simulink library "mach_lib"  (Simulink 6.3)
undefined symbols (not defined in the file): accel_cmd, aero_surf_qbar_off, aero_surf_qbar_on, altitude_stop, angular_rate_stop, att_cmd_select, att_trim_IC, att_type, att_type_numbers, bb_ellipsoid, bb_params, chi_trim_IC, command_time, compute_all_rate_cols, compute_all_vel_cols, constants, cosA, da_trim_IC, de_trim_IC, DiscIntNeverNeededParam, dr_trim_IC, dtsim, E_rwy, E_trim_IC, Ed_cmd, Ed_trim_IC, energy_stop, eow_boundary, full_surf_llim, full_surf_ulim, gain_var_struct, gam_cmd_descent, gam_cmd_preflare, gamdot_cmd_descent, gamdot_cmd_flare, gamdot_cmd_preflare, gamma_trim_IC, h_trim_IC, hd_cmd, hd_trim_IC, ideal_vel_Kb, integrate_start_time_sim, integrate_state_sim, llim, MACH, MACH_att_fb, MACH_gain_mat, MACH_mass_IC, MACH_pos_IC, MACH_pqr_Bmat_IC, MACH_pqr_IC, MACH_pqr_u_IC, MACH_quat_IC, MACH_throttle_IC, MACH_U_nom_IC, MACH_vel_Bmat_IC, MACH_vel_cvdnom_IC, MACH_vel_IC, MACH_vel_uold_IC, max_chi_cmd ... (+67)
libraries: simulink x75, mach_lib x27, utility_lib x25, model_lib x7, models x6
(part 4 of 6)

== system mach_lib/claw_main/grab ExportedGlobal/grab cv variables/Subsystem ==
  In1 : Inport
  In2 : Inport  Port=2
  In3 : Inport  Port=3
  In4 : Inport  Port=4
  In5 : Inport  Port=5
  In6 : Inport  Port=6
  In7 : Inport  Port=7
  In8 : Inport  Port=8
  In9 : Inport  Port=9
  In10 : Inport  Port=10
  In11 : Inport  Port=11
  In12 : Inport  Port=12
  In13 : Inport  Port=13
  Out1 : Outport
  Out2 : Outport  Port=2
  Out3 : Outport  Port=3
  Out4 : Outport  Port=4
  Out5 : Outport  Port=5
  Out6 : Outport  Port=6
  Out7 : Outport  Port=7
  Out8 : Outport  Port=8
  Out9 : Outport  Port=9
  Out10 : Outport  Port=10
  Out11 : Outport  Port=11
  Out12 : Outport  Port=12
  Out13 : Outport  Port=13
  wires:
  In13/1 -> Out13/1
  In12/1 -> Out12/1
  In11/1 -> Out11/1
  In10/1 -> Out10/1
  In9/1 -> Out9/1
  In8/1 -> Out8/1
  In7/1 -> Out7/1
  In6/1 -> Out6/1
  In5/1 -> Out5/1
  In4/1 -> Out4/1
  In3/1 -> Out3/1
  In2/1 -> Out2/1
  In1/1 -> Out1/1

== system mach_lib/claw_main/grab ExportedGlobal/grab cvcmd variables/Subsystem ==
  In1 : Inport
  In2 : Inport  Port=2
  In3 : Inport  Port=3
  In4 : Inport  Port=4
  In5 : Inport  Port=5
  In6 : Inport  Port=6
  In7 : Inport  Port=7
  In8 : Inport  Port=8
  In9 : Inport  Port=9
  In10 : Inport  Port=10
  In11 : Inport  Port=11
  In12 : Inport  Port=12
  In13 : Inport  Port=13
  Out1 : Outport
  Out2 : Outport  Port=2
  Out3 : Outport  Port=3
  Out4 : Outport  Port=4
  Out5 : Outport  Port=5
  Out6 : Outport  Port=6
  Out7 : Outport  Port=7
  Out8 : Outport  Port=8
  Out9 : Outport  Port=9
  Out10 : Outport  Port=10
  Out11 : Outport  Port=11
  Out12 : Outport  Port=12
  Out13 : Outport  Port=13
  wires:
  In13/1 -> Out13/1
  In12/1 -> Out12/1
  In11/1 -> Out11/1
  In10/1 -> Out10/1
  In9/1 -> Out9/1
  In8/1 -> Out8/1
  In7/1 -> Out7/1
  In6/1 -> Out6/1
  In5/1 -> Out5/1
  In4/1 -> Out4/1
  In3/1 -> Out3/1
  In2/1 -> Out2/1
  In1/1 -> Out1/1

== system mach_lib/claw_main/grab ExportedGlobal/grab cvdex variables/Subsystem ==
  In1 : Inport
  In2 : Inport  Port=2
  In3 : Inport  Port=3
  In4 : Inport  Port=4
  In5 : Inport  Port=5
  In6 : Inport  Port=6
  In7 : Inport  Port=7
  In8 : Inport  Port=8
  In9 : Inport  Port=9
  In10 : Inport  Port=10
  In11 : Inport  Port=11
  In12 : Inport  Port=12
  In13 : Inport  Port=13
  Out1 : Outport
  Out2 : Outport  Port=2
  Out3 : Outport  Port=3
  Out4 : Outport  Port=4
  Out5 : Outport  Port=5
  Out6 : Outport  Port=6
  Out7 : Outport  Port=7
  Out8 : Outport  Port=8
  Out9 : Outport  Port=9
  Out10 : Outport  Port=10
  Out11 : Outport  Port=11
  Out12 : Outport  Port=12
  Out13 : Outport  Port=13
  wires:
  In13/1 -> Out13/1
  In12/1 -> Out12/1
  In11/1 -> Out11/1
  In10/1 -> Out10/1
  In9/1 -> Out9/1
  In8/1 -> Out8/1
  In7/1 -> Out7/1
  In6/1 -> Out6/1
  In5/1 -> Out5/1
  In4/1 -> Out4/1
  In3/1 -> Out3/1
  In2/1 -> Out2/1
  In1/1 -> Out1/1

== system mach_lib/claw_main/grab ExportedGlobal/grab integrator variables/Subsystem ==
  In1 : Inport
  In2 : Inport  Port=2
  In3 : Inport  Port=3
  In4 : Inport  Port=4
  In5 : Inport  Port=5
  In6 : Inport  Port=6
  In7 : Inport  Port=7
  In8 : Inport  Port=8
  In9 : Inport  Port=9
  In10 : Inport  Port=10
  In11 : Inport  Port=11
  In12 : Inport  Port=12
  In13 : Inport  Port=13
  Out1 : Outport
  Out2 : Outport  Port=2
  Out3 : Outport  Port=3
  Out4 : Outport  Port=4
  Out5 : Outport  Port=5
  Out6 : Outport  Port=6
  Out7 : Outport  Port=7
  Out8 : Outport  Port=8
  Out9 : Outport  Port=9
  Out10 : Outport  Port=10
  Out11 : Outport  Port=11
  Out12 : Outport  Port=12
  Out13 : Outport  Port=13
  wires:
  In13/1 -> Out13/1
  In12/1 -> Out12/1
  In11/1 -> Out11/1
  In10/1 -> Out10/1
  In9/1 -> Out9/1
  In8/1 -> Out8/1
  In7/1 -> Out7/1
  In6/1 -> Out6/1
  In5/1 -> Out5/1
  In4/1 -> Out4/1
  In3/1 -> Out3/1
  In2/1 -> Out2/1
  In1/1 -> Out1/1

== system mach_lib/claw_main/grab ExportedGlobal/grab w_est variables/Subsystem ==
  In1 : Inport
  In2 : Inport  Port=2
  In3 : Inport  Port=3
  Out1 : Outport
  Out2 : Outport  Port=2
  Out3 : Outport  Port=3
  wires:
  In3/1 -> Out3/1
  In2/1 -> Out2/1
  In1/1 -> Out1/1

== system mach_lib/claw_main/input processing/mode dependent stick processing/att rate cmd ==
  note: In attitude, velocity, position mode, while enabled,
      | replace cam command with integrated rate command.
      |
      | In attitude mode, while enabled,
      | replace the other att commands with integrated rate commands.
      |
      | integrators are set to current values upon transition into this condition.
      | Reset of cam cmd can be disabled by setting
      | reset_camcmd_on_entry to false.
      |
      | In addition to specified conditions, reset also occurs, if applicable
      | when att_type changes
  mode : Inport
  command_in : Inport  Port=2
  signal_bus : Inport  Port=3
  Bus Selector3 : BusSelector  OutputSignals=mode_sw.att_rate_cmd_sw,mode_sw.cam_rate_cmd_sw,y_meas.dircos
  Compare To Constant1 : simulink/Logic and Bit Operations/Compare To Constant  relop===  const=modes.att  LogicOutDataTypeMode=boolean  ZeroCross=off
  Compare To Constant2 : simulink/Logic and Bit Operations/Compare To Constant  relop=>=  const=modes.att  LogicOutDataTypeMode=boolean  ZeroCross=off
  Gain1 : Gain  Gain=[ 1 1 reset_camcmd_on_entry ]
  Logical Operator1 : Logic  Operator=OR  AllPortsSameDT=off
  Logical Operator2 : Logic  AllPortsSameDT=off
  Logical Operator4 : Logic  AllPortsSameDT=off
  Multiport Switch1 : MultiPortSwitch  Inputs=2  zeroidx=on
  Mux : Mux  Inputs=3
  Product1 : Product  RndMeth=Zero
  also reset att on att_type change : Subsystem
  att cmd integration : DiscreteIntegrator  ExternalReset=either  InitialConditionSource=external  SampleTime=-1  ICPrevOutput=DiscIntNeverNeededParam  ICPrevScaledInput=DiscIntNeverNeededParam
  att/att rate cmd : Selector  Elements=1:3  InputPortWidth=4
  dc2att : utility_lib/dc2att
  set att cmd : Assignment  Elements=1:3  OutputInitialize=Initialize using input (U1)
  command_out : Outport
  wires:
  Bus Selector3/3 -> dc2att/1  "<dircos>"
  Bus Selector3/2 -> Logical Operator1/2  "<cam_rate_cmd_sw>"
  Bus Selector3/1 -> Logical Operator1/1, Logical Operator4/2  "<att_rate_cmd_sw>"
  signal_bus/1 -> Bus Selector3/1
  dc2att/1 -> att cmd integration/3
  set att cmd/1 -> command_out/1
  Multiport Switch1/1 -> set att cmd/2
  Mux/1 -> Multiport Switch1/1, also reset att on att_type change/1(reset_in), Product1/2
  Compare To Constant2/1 -> Logical Operator2/2
  Logical Operator2/1 -> Mux/3
  Logical Operator1/1 -> Logical Operator2/1
  Logical Operator4/1 -> Mux/2, Mux/1
  att/att rate cmd/1 -> Multiport Switch1/2, Product1/1
  Compare To Constant1/1 -> Logical Operator4/1
  command_in/1 -> att/att rate cmd/1, set att cmd/1
  mode/1 -> Compare To Constant2/1, Compare To Constant1/1
  also reset att on att_type change/1(reset_out) -> Gain1/1
  att cmd integration/1 -> Multiport Switch1/3
  Gain1/1 -> att cmd integration/2
  Product1/1 -> att cmd integration/1

== system mach_lib/claw_main/input processing/mode dependent stick processing/att_type cmd ==
  mode : Inport
  command_in : Inport  Port=2
  signal_bus : Inport  Port=3
  Bus Selector3 : BusSelector  OutputSignals=mode_sw.att_type
  Compare To Constant1 : simulink/Logic and Bit Operations/Compare To Constant  relop===  const=modes.att  LogicOutDataTypeMode=boolean  ZeroCross=off
  Constant4 : Constant  Value=use_auto_att_type
  From Workspace1 : FromWorkspace  VariableName=rpy_cmd_fw  SampleTime=MACH.dt  OutputAfterFinalValue=Holding final value
  From Workspace2 : FromWorkspace  VariableName=mab_cmd_fw  SampleTime=MACH.dt  OutputAfterFinalValue=Holding final value
  From Workspace4 : FromWorkspace  VariableName=tiltcam_cmd_fw  SampleTime=MACH.dt  OutputAfterFinalValue=Holding final value
  Logical Operator4 : Logic  AllPortsSameDT=off
  Multiport Switch1 : MultiPortSwitch  Inputs=2  zeroidx=on
  Multiport Switch2 : MultiPortSwitch  Inputs=length(att_type_numbers)
  att cmd : Selector  Elements=1:3  InputPortWidth=4
  bam_cmd : Selector  Elements=[3 2 1]  InputPortWidth=3
  set att cmd : Assignment  Elements=1:3  OutputInitialize=Initialize using input (U1)
  ypr_cmd : Selector  Elements=[3 2 1]  InputPortWidth=3
  command_out : Outport
  wires:
  ypr_cmd/1 -> Multiport Switch2/4
  Multiport Switch2/1 -> Multiport Switch1/3
  bam_cmd/1 -> Multiport Switch2/6
  From Workspace1/1 -> ypr_cmd/1, Multiport Switch2/3
  From Workspace2/1 -> bam_cmd/1, Multiport Switch2/5
  From Workspace4/1 -> Multiport Switch2/2
  Bus Selector3/1 -> Multiport Switch2/1  "<att_type>"
  Constant4/1 -> Logical Operator4/2
  mode/1 -> Compare To Constant1/1
  command_in/1 -> set att cmd/1, att cmd/1
  Compare To Constant1/1 -> Logical Operator4/1
  att cmd/1 -> Multiport Switch1/2
  Logical Operator4/1 -> Multiport Switch1/1
  Multiport Switch1/1 -> set att cmd/2
  set att cmd/1 -> command_out/1
  signal_bus/1 -> Bus Selector3/1

== system mach_lib/claw_main/input processing/mode dependent stick processing/feed forward ==
  table_bus : Inport
  signal_bus : Inport  Port=2
  Bus Creator : BusCreator
  Bus Selector : BusSelector  OutputSignals=eow_idx,eow_large,X_idx
  Constant : Constant  Value=use_eow_as_iv
  Constant1 : Constant  Value=zeros(MACH.pqr_num_cv,1)
  From Workspace1 : FromWorkspace  VariableName=vel_ff_fw  SampleTime=MACH.dt  OutputAfterFinalValue=Holding final value
  From Workspace4 : FromWorkspace  VariableName=pos_ff_fw  SampleTime=MACH.dt  OutputAfterFinalValue=Holding final value
  Switch{,1..3} (4 alike) : Switch  Threshold=0.5
  get att_ff : Subsystem
  lookup using  energy over weight : Subsystem
  "lookup using X  " : Subsystem
  feed_forward : Outport
  wires:
  signal_bus/1 -> get att_ff/1(signal_bus)
  Bus Selector/3 -> "lookup using X  "/1(X_idx)  "<X_idx>"
  Bus Selector/2 -> Switch3/2, Switch2/2  "<eow_large>"
  Bus Selector/1 -> lookup using  energy over weight/1(eow_idx)  "<eow_idx>"
  table_bus/1 -> Bus Selector/1
  "lookup using X  "/1(pos_ff) -> Switch2/3
  "lookup using X  "/2(vel_ff) -> Switch3/3
  lookup using  energy over weight/2(vel_ff) -> Switch3/1
  Switch3/1 -> Switch1/1
  lookup using  energy over weight/1(pos_ff) -> Switch2/1
  Switch2/1 -> Switch/1
  Constant/1 -> Switch/2, Switch1/2
  From Workspace1/1 -> Switch1/3
  From Workspace4/1 -> Switch/3
  Bus Creator/1 -> feed_forward/1
  Constant1/1 -> Bus Creator/4  "pqr_ff"
  get att_ff/1(att_ff) -> Bus Creator/3  "att_ff"
  Switch1/1 -> Bus Creator/2  "vel_ff"
  Switch/1 -> Bus Creator/1  "pos_ff"

== system mach_lib/claw_main/input processing/mode dependent stick processing/llh cmd ==
  mode : Inport
  command_in : Inport  Port=2
  signal_bus : Inport  Port=3
  Assignment : Assignment  Elements=[1 2 4]  OutputInitialize=Initialize using input (U1)
  Bus Selector : BusSelector  OutputSignals=mode_sw.llh_input_sw,y_meas.vehicle_origin
  Compare To Constant1 : simulink/Logic and Bit Operations/Compare To Constant  relop===  const=modes.pos  LogicOutDataTypeMode=boolean  ZeroCross=off
  LLh2NEh : utility_lib/LLh2NEh
  Logical Operator4 : Logic  AllPortsSameDT=off
  Multiport Switch2 : MultiPortSwitch  Inputs=2  zeroidx=on  SaturateOnIntegerOverflow=on
  Selector1 : Selector  Elements=[1 2 4]  InputPortWidth=4
  command_out : Outport
  wires:
  mode/1 -> Compare To Constant1/1
  Logical Operator4/1 -> Multiport Switch2/1
  Bus Selector/1 -> Logical Operator4/2  "<llh_input_sw>"
  Compare To Constant1/1 -> Logical Operator4/1
  signal_bus/1 -> Bus Selector/1
  Multiport Switch2/1 -> command_out/1
  Assignment/1 -> Multiport Switch2/3
  LLh2NEh/1 -> Assignment/2
  Selector1/1 -> LLh2NEh/1
  command_in/1 -> Selector1/1, Assignment/1, Multiport Switch2/2
  Bus Selector/2 -> LLh2NEh/2  "<vehicle_origin>"

== system mach_lib/claw_main/input processing/mode dependent stick processing/rampin vel_cmd ==
  mode : Inport
  command_in : Inport  Port=2
  NEh_dot : Inport  Port=3
  Compare To Constant : simulink/Logic and Bit Operations/Compare To Constant  relop=<=  const=modes.att  LogicOutDataTypeMode=boolean  ZeroCross=off
  Compare To Constant1 : simulink/Logic and Bit Operations/Compare To Constant  relop===  const=modes.vel  LogicOutDataTypeMode=boolean  ZeroCross=off
  Constant : Constant  Value=MACH.dt/max(vel_cmd_ramp_time,MACH.dt)
  Constant1 : Constant
  Constant2 : Constant  Value=0
  Logical Operator : Logic  AllPortsSameDT=off
  MinMax : MinMax  Function=max  Inputs=2
  Product : Product  RndMeth=Zero
  Product1 : Product  RndMeth=Zero
  Sum : Sum  Inputs=-+|
  Sum2 : Sum  Inputs=|++
  Sum3 : Sum  Inputs=|+-
  Switch : Switch  Threshold=0.5
  Switch1 : Switch  Threshold=0.5
  Unit Delay : UnitDelay  Orientation=left  SampleTime=-1
  Unit Delay1 : UnitDelay  SampleTime=-1
  Unit Delay2 : UnitDelay  Orientation=left  SampleTime=-1
  set vel cmd : Assignment  Elements=[1 2 4]  OutputInitialize=Initialize using input (U1)
  vel cmd : Selector  Elements=[1 2 4]  InputPortWidth=4
  command_out : Outport
  wires:
  Constant2/1 -> MinMax/1
  MinMax/1 -> Unit Delay2/1, Product/2
  Constant/1 -> Sum3/2
  Sum3/1 -> MinMax/2
  Product/1 -> Sum2/2
  Switch1/1 -> Sum3/1
  Constant1/1 -> Switch1/1
  Product1/1 -> Switch1/3
  Sum2/1 -> set vel cmd/2
  command_in/1 -> vel cmd/1, set vel cmd/1
  vel cmd/1 -> Sum/1, Sum2/1
  set vel cmd/1 -> command_out/1
  Sum/1 -> Switch/1
  NEh_dot/1 -> Sum/2
  Switch/1 -> Product/1, Unit Delay/1
  Unit Delay/1 -> Switch/3
  mode/1 -> Compare To Constant1/1, Unit Delay1/1
  Unit Delay1/1 -> Compare To Constant/1
  Compare To Constant/1 -> Logical Operator/1
  Compare To Constant1/1 -> Product1/1, Logical Operator/2
  Logical Operator/1 -> Switch1/2, Switch/2
  Unit Delay2/1 -> Product1/2

== system mach_lib/claw_main/input processing/mode dependent stick processing/set command selection switches ==
  accel_cmd_sw : Inport
  CLAW_mode : Inport  Port=2
  Bus Creator : BusCreator
  Constant : Constant  Value=MACH.select_cmd_array
  Demux : Demux  Outputs=[4 5 4 4]
  Reshape : simulink/Math Operations/Reshape  OutputDimensionality=1-D array  OutputDimensions=[1,1]
  Selector : Selector  InputType=Matrix  IndexMode=Zero-based  Elements=[1 3]  Rows=-1  ColumnSrc=External  InputPortWidth=3
  modify for accel cmd submode : Subsystem
  select_cmd : Outport
  wires:
  accel_cmd_sw/1 -> modify for accel cmd submode/2(accel_cmd_sw)
  Bus Creator/1 -> modify for accel cmd submode/1(select_cmd_in)
  modify for accel cmd submode/1(select_cmd) -> select_cmd/1
  Reshape/1 -> Demux/1
  Demux/4 -> Bus Creator/4  "pos"
  Demux/3 -> Bus Creator/3  "vel"
  Demux/2 -> Bus Creator/2  "att"
  Demux/1 -> Bus Creator/1  "rate"
  Selector/1 -> Reshape/1
  CLAW_mode/1 -> Selector/2
  Constant/1 -> Selector/1

== system mach_lib/claw_main/input processing/mode dependent stick processing/table iv computation ==
  x_est : Inport
  Bus Creator : BusCreator  Inputs=5
  Compare To Constant : simulink/Logic and Bit Operations/Compare To Constant  relop=>=  const=eow_boundary  LogicOutDataTypeMode=boolean  ZeroCross=off
  Constant : Constant  Value=2*constants.g
  Constant1 : Constant  Value=sinA
  Constant2 : Constant  Value=cosA
  Constant3 : Constant  Value=N_rwy
  Constant4 : Constant  Value=E_rwy
  Dot Product : simulink/Math Operations/Dot Product  InputSameDT=on  OutDataType=sfix(16)  OutScaling=2^-10  DoSatur=off
  PreLookup Index Search : simulink/Lookup Tables/PreLookup Index Search  bpData=tbl_eow  searchMode=Binary Search  cacheBpFlag=off  outputFlag=off  IndexDataType=uint32  extrapMode=Linear Extrapolation  rangeErrorMode=None
  PreLookup Index Search1 : simulink/Lookup Tables/PreLookup Index Search  bpData=tbl_X  searchMode=Binary Search  cacheBpFlag=off  outputFlag=off  IndexDataType=uint32  extrapMode=Clip to Range  rangeErrorMode=None
  Product1 : Product  RndMeth=Zero
  Product2 : Product  Inputs=*/  RndMeth=Zero
  Product3 : Product  RndMeth=Zero
  Sum1 : Sum  Inputs=|++
  Sum2 : Sum  Inputs=-+|
  Sum3 : Sum  Inputs=+|+
  Sum4 : Sum  Inputs=|+-
  get E : Selector  Elements=8  InputPortWidth=13
  get N : Selector  Elements=7  InputPortWidth=13
  get h : Selector  Elements=9  InputPortWidth=13
  get uvw : Selector  Elements=4:6  InputPortWidth=13
  table_bus : Outport
  wires:
  Compare To Constant/1 -> Bus Creator/1  "eow_large"
  PreLookup Index Search1/1 -> Bus Creator/5  "X_idx"
  Bus Creator/1 -> table_bus/1
  Sum3/1 -> Bus Creator/4, PreLookup Index Search1/1  "X"
  Sum4/1 -> Product1/2
  Constant4/1 -> Sum4/2
  Constant3/1 -> Sum2/1
  Constant1/1 -> Product1/1
  Product1/1 -> Sum3/2
  get E/1 -> Sum4/1
  Constant2/1 -> Product3/2
  Product3/1 -> Sum3/1
  Sum2/1 -> Product3/1
  get N/1 -> Sum2/2
  PreLookup Index Search/1 -> Bus Creator/3  "eow_idx"
  Sum1/1 -> Bus Creator/2, Compare To Constant/1, PreLookup Index Search/1  "eow"
  x_est/1 -> get E/1, get N/1, get uvw/1, get h/1
  Product2/1 -> Sum1/2
  Dot Product/1 -> Product2/1
  Constant/1 -> Product2/2
  get h/1 -> Sum1/1
  get uvw/1 -> Dot Product/2, Dot Product/1

== system mach_lib/claw_main/input processing/mode dependent stick processing/use table lookup pos cmds ==
  mode : Inport
  command_in : Inport  Port=2
  table_bus : Inport  Port=3
  Assertion : Assertion  Enabled=off  AssertionFailFcn=assertioncb  StopWhenAssertionFail=off
  Bus Selector : BusSelector  OutputSignals=eow_idx,eow_large,X_idx,X
  Compare To Constant1 : simulink/Logic and Bit Operations/Compare To Constant  relop===  const=modes.pos  LogicOutDataTypeMode=boolean  ZeroCross=off
  Constant4 : Constant  Value=use_eow_as_iv
  Logical Operator : Logic  AllPortsSameDT=off
  Relational Operator : RelationalOperator  LogicOutDataTypeMode=Boolean
  Switch1 : Switch  Threshold=0.5
  Switch2 : Switch  Threshold=0.5
  Unit Delay : UnitDelay  SampleTime=-1
  pos cmd : Selector  Elements=[1 2 4]  InputPortWidth=4
  set pos cmd : Assignment  Elements=[1 2 4]  OutputInitialize=Initialize using input (U1)
  use E/W to get pos cmds : Subsystem
  use X to get pos cmds : Subsystem
  command_out : Outport
  wires:
  Relational Operator/1 -> Assertion/1
  Unit Delay/1 -> Relational Operator/1
  Bus Selector/4 -> use X to get pos cmds/2(X)  "<X>"
  Bus Selector/3 -> use X to get pos cmds/1(X_idx)  "<X_idx>"
  Bus Selector/1 -> use E/W to get pos cmds/1(eow_idx)  "<eow_idx>"
  table_bus/1 -> Bus Selector/1
  Bus Selector/2 -> Switch1/2  "<eow_large>"
  Switch1/1 -> Switch2/1
  use X to get pos cmds/1(pos_cmd_X) -> Switch1/3
  use E/W to get pos cmds/1(pos_cmd_eow) -> Switch1/1
  Switch2/1 -> set pos cmd/2
  command_in/1 -> pos cmd/1, set pos cmd/1
  pos cmd/1 -> Switch2/3
  set pos cmd/1 -> command_out/1
  mode/1 -> Compare To Constant1/1
  Constant4/1 -> Logical Operator/1
  Compare To Constant1/1 -> Logical Operator/2
  Logical Operator/1 -> Relational Operator/2, Unit Delay/1, Switch2/2

== system mach_lib/claw_main/input processing/modify limits and apply to direct commands/apply surface locking ==
  u_meas : Inport
  full_surf_in : Inport  Port=2
  Bus Assignment : BusAssignment  AssignedSignals=full_surf_ulim,full_surf_llim
  Bus Selector : BusSelector  OutputSignals=full_surf_ulim,full_surf_cmd,full_surf_lock,full_surf_llim
  Multiport Switch : MultiPortSwitch  Inputs=3  zeroidx=on
  Multiport Switch1 : MultiPortSwitch  Inputs=3  zeroidx=on
  full_surf : Outport
  wires:
  Bus Selector/4 -> Multiport Switch1/2  "<full_surf_llim>"
  Bus Selector/2 -> Multiport Switch1/3, Multiport Switch/3  "<full_surf_cmd>"
  Bus Selector/1 -> Multiport Switch/2  "<full_surf_ulim>"
  Bus Selector/3 -> Multiport Switch/1, Multiport Switch1/1  "<full_surf_lock>"
  Bus Assignment/1 -> full_surf/1
  u_meas/1 -> Multiport Switch/4, Multiport Switch1/4
  Multiport Switch1/1 -> Bus Assignment/3
  Multiport Switch/1 -> Bus Assignment/2
  full_surf_in/1 -> Bus Assignment/1, Bus Selector/1

== system mach_lib/claw_main/input processing/modify limits and apply to direct commands/throt out of fuel limits ==
  full_surf_in : Inport
  Bus Assignment : BusAssignment  AssignedSignals=full_surf_ulim,full_surf_llim
  Bus Selector3 : BusSelector  OutputSignals=full_surf_ulim,full_surf_llim
  throt out of fuel limits : model_lib/throt out of fuel limits
  full_surf : Outport
  wires:
  throt out of fuel limits/2 -> Bus Assignment/3
  throt out of fuel limits/1 -> Bus Assignment/2
  Bus Assignment/1 -> full_surf/1
  full_surf_in/1 -> Bus Assignment/1, Bus Selector3/1
  Bus Selector3/2 -> throt out of fuel limits/2  "<full_surf_llim>"
  Bus Selector3/1 -> throt out of fuel limits/1  "<full_surf_ulim>"

== system mach_lib/claw_main/input processing/select att_type/add tiebreaker for current att_type ==
  att_type_selected : Inport
  priority_in : Inport  Port=2
  Assignment1 : Assignment  IndexMode=Zero-based  ElementSrc=External  OutputInitialize=Initialize using input (U1)  OutputDimensions=length(att_type_numbers)+1
  Constant1 : Constant  Value=0.5
  Selector : Selector  IndexMode=Zero-based  ElementSrc=External  Elements=[1 3]  InputPortWidth=length(att_type_numbers)+1
  Sum1 : Sum  Inputs=|++
  Unit Delay : UnitDelay  SampleTime=-1
  priority_out : Outport
  wires:
  Assignment1/1 -> priority_out/1
  Unit Delay/1 -> Assignment1/3, Selector/2
  Sum1/1 -> Assignment1/2
  Constant1/1 -> Sum1/2
  Selector/1 -> Sum1/1
  priority_in/1 -> Assignment1/1, Selector/1
  att_type_selected/1 -> Unit Delay/1

== system mach_lib/claw_main/input processing/select att_type/compute precond vars ==
  signal_bus : Inport
  scoped_bus : Inport  Port=2
  -sin_b : Selector  InputPortWidth=9
  -sin_theta : Selector  Elements=7  InputPortWidth=9
  Bus Creator : BusCreator  Inputs=6
  Bus Selector2 : BusSelector  OutputSignals=aero_env_est.qbar,aero_env_est.vel,aero_env_est.beta,y_meas.dircos
  Bus Selector4 : BusSelector  OutputSignals=dc_L2W
  Saturation : Saturate  UpperLimit=1  LowerLimit=-1
  Saturation1 : Saturate  UpperLimit=1  LowerLimit=-1
  Trigonometric Function : Trigonometry  Operator=cos
  abs_cos_b : Fcn  Expr=sqrt(1-u(1)^2)
  abs_cos_beta : Abs
  abs_cos_gamma_rw : Abs
  abs_cos_theta : Fcn  Expr=sqrt(1-u(1)^2)
  abs_vel_rw : Abs
  cos_gamma_rw : Selector  Elements=9  InputPortWidth=9
  precond_vars : Outport
  wires:
  scoped_bus/1 -> Bus Selector4/1
  Bus Creator/1 -> precond_vars/1
  signal_bus/1 -> Bus Selector2/1
  Saturation1/1 -> abs_cos_b/1
  Saturation/1 -> abs_cos_theta/1
  abs_cos_gamma_rw/1 -> Bus Creator/6  "abs_cos_gamma_rw"
  abs_cos_b/1 -> Bus Creator/5  "abs_cos_b"
  abs_cos_theta/1 -> Bus Creator/4  "abs_cos_theta"
  abs_cos_beta/1 -> Bus Creator/3  "abs_cos_beta"
  abs_vel_rw/1 -> Bus Creator/2  "abs_vel_rw"
  cos_gamma_rw/1 -> abs_cos_gamma_rw/1
  -sin_theta/1 -> Saturation/1
  -sin_b/1 -> Saturation1/1
  Trigonometric Function/1 -> abs_cos_beta/1
  Bus Selector2/4 -> -sin_b/1, -sin_theta/1  "<dircos>"
  Bus Selector2/3 -> Trigonometric Function/1  "<beta>"
  Bus Selector2/2 -> abs_vel_rw/1  "<vel>"
  Bus Selector2/1 -> Bus Creator/1  "<qbar>"
  Bus Selector4/1 -> cos_gamma_rw/1  "<dc_L2W>"

== system mach_lib/claw_main/input processing/select att_type/evaluate preconditions ==
  precond_vars : Inport
  Bus Selector5 : BusSelector  OutputSignals=abs_cos_b,abs_cos_theta,abs_vel_rw,abs_cos_beta,abs_cos_gamma_rw,qbar
  Compare To Constant : simulink/Logic and Bit Operations/Compare To Constant  relop=>=  const=1  LogicOutDataTypeMode=boolean  ZeroCross=off
  Compare To Constant1 : simulink/Logic and Bit Operations/Compare To Constant  relop=>=  const=cos(pi/3)  LogicOutDataTypeMode=boolean  ZeroCross=off
  Compare To Constant2 : simulink/Logic and Bit Operations/Compare To Constant  relop=>=  const=0.1  LogicOutDataTypeMode=boolean  ZeroCross=off
  Compare To Constant3 : simulink/Logic and Bit Operations/Compare To Constant  relop=>=  const=cos(pi/3)  LogicOutDataTypeMode=boolean  ZeroCross=off
  Compare To Constant4 : simulink/Logic and Bit Operations/Compare To Constant  relop=>=  const=cos(pi/3)  LogicOutDataTypeMode=boolean  ZeroCross=off
  Compare To Constant5 : simulink/Logic and Bit Operations/Compare To Constant  relop=>=  const=1  LogicOutDataTypeMode=boolean  ZeroCross=off
  Constant : Constant  Value=boolean(0)
  Logical Operator : Logic  Inputs=4  AllPortsSameDT=off  OutDataTypeMode=Boolean
  Mux : Mux  Inputs=6
  precond_satisfied : Outport
  wires:
  Mux/1 -> precond_satisfied/1
  precond_vars/1 -> Bus Selector5/1
  Bus Selector5/6 -> Compare To Constant5/1  "<qbar>"
  Compare To Constant5/1 -> Logical Operator/4
  Constant/1 -> Mux/1
  Logical Operator/1 -> Mux/6, Mux/5
  Bus Selector5/5 -> Compare To Constant2/1  "<abs_cos_gamma_rw>"
  Bus Selector5/4 -> Compare To Constant1/1  "<abs_cos_beta>"
  Bus Selector5/3 -> Compare To Constant/1  "<abs_vel_rw>"
  Bus Selector5/2 -> Compare To Constant3/1  "<abs_cos_theta>"
  Bus Selector5/1 -> Compare To Constant4/1  "<abs_cos_b>"
  Compare To Constant4/1 -> Mux/2
  Compare To Constant3/1 -> Mux/4, Mux/3
  Compare To Constant2/1 -> Logical Operator/3
  Compare To Constant1/1 -> Logical Operator/2
  Compare To Constant/1 -> Logical Operator/1

== system mach_lib/claw_main/input processing/select att_type/select best att_type ==
  vec : Inport
  Constant4 : Constant  Value=0:length(att_type_numbers)
  Constant5 : Constant  Value=length(att_type_numbers)
  MinMax3 : MinMax  Function=max  SaturateOnIntegerOverflow=on  InputSameDT=on
  MinMax4 : MinMax  SaturateOnIntegerOverflow=on  InputSameDT=on
  Sum2 : Sum  Inputs=+-|  SaturateOnIntegerOverflow=on
  argmax1 : Switch  Threshold=-eps  SaturateOnIntegerOverflow=on
  idx_max : Outport
  wires:
  MinMax4/1 -> idx_max/1
  MinMax3/1 -> Sum2/2
  argmax1/1 -> MinMax4/1
  Constant5/1 -> argmax1/3
  Constant4/1 -> argmax1/1
  Sum2/1 -> argmax1/2
  vec/1 -> Sum2/1, MinMax3/1

== system mach_lib/claw_main/input processing/set control parameters/accel submode setup ==
  signal_bus : Inport
  Bus Selector1 : BusSelector  OutputSignals=mode_sw.enable_homing_sw,mode_sw.accel_submode,mode_sw.CLAW_mode
  Constant1 : Constant  Value=3
  Constant2 : Constant  Value=0
  Merge1 : Merge  Inputs=3  InitialOutput=zeros(3,1)
  Merge2 : Merge  Inputs=3  InitialOutput=zeros(3,1)
  NED_dd/vchigam_dot : Subsystem  TreatAsAtomicUnit=on
  Switch : Switch  Threshold=0.5
  Switch Case : SwitchCase  CaseConditions={[1 2],3}
  Switch1 : Switch  Threshold=0.5  InputSameDT=on
  homing : Subsystem  TreatAsAtomicUnit=on
  normal vel desdyn : Subsystem  TreatAsAtomicUnit=on
  accel_cmd_sw : Outport
  accel_cmd : Outport  Port=2
  wires:
  signal_bus/1 -> homing/1(signal_bus), NED_dd/vchigam_dot/2(signal_bus), Bus Selector1/1
  Constant2/1 -> Switch1/3
  Bus Selector1/3 -> Switch1/2  "<CLAW_mode>"
  normal vel desdyn/1(accel_cmd_sw) -> Merge2/3
  homing/1(accel_cmd_sw) -> Merge2/2
  homing/2(accel_cmd) -> Merge1/2
  NED_dd/vchigam_dot/2(accel_cmd) -> Merge1/1
  normal vel desdyn/2(accel_cmd) -> Merge1/3
  NED_dd/vchigam_dot/1(accel_cmd_sw) -> Merge2/1
  Merge2/1 -> accel_cmd_sw/1
  Merge1/1 -> accel_cmd/1
  Switch Case/3 -> normal vel desdyn/Action
  Switch Case/2 -> homing/Action
  Switch Case/1 -> NED_dd/vchigam_dot/Action
  Switch1/1 -> NED_dd/vchigam_dot/1(case), Switch Case/1
  Switch/1 -> Switch1/1
  Bus Selector1/2 -> Switch/3  "<accel_submode>"
  Bus Selector1/1 -> Switch/2  "<enable_homing_sw>"
  Constant1/1 -> Switch/1

== system mach_lib/claw_main/input processing/set control parameters/modify MACH_att_Kf ==
  gain_bus_in : Inport
  signal_bus : Inport  Port=2
  Bus Assignment : BusAssignment  AssignedSignals=MACH_att_Kf
  Bus Selector : BusSelector  OutputSignals=mode_sw.att_type
  Bus Selector1 : BusSelector  OutputSignals=MACH_att_Kf
  Compare To Constant : simulink/Logic and Bit Operations/Compare To Constant  relop=>=  const=att_type.mba_bank  LogicOutDataTypeMode=boolean  ZeroCross=off
  Constant : Constant  Value=MACH_att_fb
  Logical Operator : Logic  AllPortsSameDT=off
  Logical Operator1 : Logic  Operator=OR  AllPortsSameDT=off  OutDataTypeMode=Boolean
  Logical Operator2 : Logic  Operator=NOT  AllPortsSameDT=off  OutDataTypeMode=Boolean
  Logical Operator3 : Logic  AllPortsSameDT=off  OutDataTypeMode=Boolean
  gain_bus : Outport
  wires:
  Bus Assignment/1 -> gain_bus/1
  Logical Operator/1 -> Bus Assignment/2
  Logical Operator1/1 -> Logical Operator/2
  Compare To Constant/1 -> Logical Operator3/2
  Logical Operator3/1 -> Logical Operator1/2
  Bus Selector/1 -> Compare To Constant/1  "<att_type>"
  signal_bus/1 -> Bus Selector/1
  gain_bus_in/1 -> Bus Selector1/1, Bus Assignment/1
  Logical Operator2/1 -> Logical Operator1/1
  Constant/1 -> Logical Operator3/1, Logical Operator2/1
  Bus Selector1/1 -> Logical Operator/1  "<MACH_att_Kf>"

== system mach_lib/claw_main/input processing/set control parameters/select gains ==
  note: Note: Current variable gain structure will use gain_set = 1
      | if it exists, when enable_bb is true, otherwise gain_set = 0
      | (which is the global or selected default)
  enable_bb : Inport
  gain_set_in : Inport  Port=2
  Constant2 : Constant  Value=MACH_gain_mat
  MinMax : MinMax  Inputs=2
  Product : Product  Inputs=*/  RndMeth=Zero
  Reshape : simulink/Math Operations/Reshape  OutputDimensionality=1-D array  OutputDimensions=[1,1]
  Switch : Switch
  Width1 : Width
  Width2 : Width
  mux to bus : Subsystem  mask{var_struct=gain_var_struct}
      mask prompts: var_struct "var struct"
      mask init:
      | if(~isstruct(var_struct) || length(var_struct) == 0 || ~isfield(var_struct,'name') || ~isfield(var_struct,'size'))
      |     error('var struct must be at least size 1, and must have the ''name'' and ''size'' fields defined.');
      | end
      | 
      | var_name = {var_struct.name};
      | var_size = prod(vertcat(var_struct.size),2);
      | nvar = length(var_name);
      | 
      | % remove old lines
      | nvar_old = length(get_param([gcb '/Demux'],'Outputs'));
      | for i = 1:nvar_old
      |     try
      |         delete_line(gcb,['Demux/' num2str(i)] ,['Bus Creator/' num2str(i)])
      |     end
      | end
      | 
      | set_param([gcb '/Demux'],'Outputs',mat2str(var_size));
      | set_param([gcb '/Bus Creator'],'Inputs',num2str(nvar));
      | port_handle = getfield(get_param([gcb '/Demux'],'PortHandles'),'Outport');
      | for i = 1:nvar
      |     try
      |         add_line(gcb,['Demux/' num2str(i)] ,['Bus Creator/' num2str(i)])
      |     end
      |     set(port_handle(i),'Name',var_name{i});
      | end
  select gain set : Selector  InputType=Matrix  IndexMode=Zero-based  Elements=[1 3]  RowSrc=External  Rows=gain_set  Columns=-1  InputPortWidth=3
  gain_set : Outport
  gain_bus : Outport  Port=2
  wires:
  Product/1 -> MinMax/2
  Switch/1 -> MinMax/1
  gain_set_in/1 -> Switch/2, Switch/1
  Width1/1 -> Product/2
  Width2/1 -> Product/1
  mux to bus/1(bus_out) -> gain_bus/1
  enable_bb/1 -> Switch/3
  MinMax/1 -> select gain set/2, gain_set/1
  Reshape/1 -> Width1/1, mux to bus/1(mux_in)
  select gain set/1 -> Reshape/1
  Constant2/1 -> Width2/1, select gain set/1

== system mach_lib/claw_main/input processing/set control parameters/set att desdyn params ==
  gain_bus : Inport
  Bus Creator : BusCreator  Inputs=7
  Bus Selector : BusSelector  OutputSignals=MACH_att_Kb,MACH_att_Ki,MACH_att_Kaw,MACH_att_Kf
  Constant1 : Constant  Value=zeros(1,4)
  Constant6 : Constant  Value=MACH_quat_IC
  Signal Specification : SignalSpecification
  Signal Specification1 : SignalSpecification
  Signal Specification2 : SignalSpecification
  compute dependent gains : mach_lib/compute dependent gains
  params : Outport
  wires:
  Constant1/1 -> compute dependent gains/6
  Constant6/1 -> compute dependent gains/5
  Signal Specification2/1 -> Bus Creator/7  "kf"
  Signal Specification1/1 -> compute dependent gains/1, Bus Creator/2  "ki"
  Signal Specification/1 -> compute dependent gains/2, Bus Creator/1  "kb"
  gain_bus/1 -> Bus Selector/1
  Bus Selector/4 -> compute dependent gains/4, Signal Specification2/1  "<MACH_att_Kf>"
  compute dependent gains/3 -> Bus Creator/5  "kaw"
  Bus Selector/2 -> Signal Specification1/1  "<MACH_att_Ki>"
  Bus Selector/1 -> Signal Specification/1  "<MACH_att_Kb>"
  Bus Creator/1 -> params/1
  compute dependent gains/1 -> Bus Creator/3  "kc"
  compute dependent gains/2 -> Bus Creator/4  "ki_trim"
  Bus Selector/3 -> compute dependent gains/3  "<MACH_att_Kaw>"
  compute dependent gains/4 -> Bus Creator/6  "x0"

== system mach_lib/claw_main/input processing/set control parameters/set pos desdyn params ==
  gain_bus : Inport
  Bus Creator : BusCreator  Inputs=7
  Bus Selector : BusSelector  OutputSignals=MACH_pos_Kb,MACH_pos_Ki,MACH_pos_Kaw,MACH_pos_Kf
  Constant3 : Constant  Value=MACH_vel_IC
  Constant6 : Constant  Value=MACH_pos_IC
  Signal Specification : SignalSpecification
  Signal Specification1 : SignalSpecification
  Signal Specification2 : SignalSpecification
  compute dependent gains : mach_lib/compute dependent gains
  params : Outport
  wires:
  Constant3/1 -> compute dependent gains/6
  Constant6/1 -> compute dependent gains/5
  Signal Specification2/1 -> Bus Creator/7  "kf"
  Signal Specification1/1 -> Bus Creator/2, compute dependent gains/1  "ki"
  Signal Specification/1 -> compute dependent gains/2, Bus Creator/1  "kb"
  gain_bus/1 -> Bus Selector/1
  compute dependent gains/4 -> Bus Creator/6  "x0"
  Bus Selector/4 -> compute dependent gains/4, Signal Specification2/1  "<MACH_pos_Kf>"
  compute dependent gains/3 -> Bus Creator/5  "kaw"
  Bus Selector/2 -> Signal Specification1/1  "<MACH_pos_Ki>"
  Bus Selector/1 -> Signal Specification/1  "<MACH_pos_Kb>"
  Bus Creator/1 -> params/1
  compute dependent gains/1 -> Bus Creator/3  "kc"
  compute dependent gains/2 -> Bus Creator/4  "ki_trim"
  Bus Selector/3 -> compute dependent gains/3  "<MACH_pos_Kaw>"

== system mach_lib/claw_main/input processing/set control parameters/set rate desdyn params ==
  gain_bus : Inport
  Bus Creator : BusCreator  Inputs=7
  Bus Selector : BusSelector  OutputSignals=MACH_pqr_Kb,MACH_pqr_Ki,MACH_pqr_Kaw,MACH_pqr_Kf
  Constant1 : Constant  Value=zeros(1,3)
  Constant6 : Constant  Value=MACH_pqr_IC
  Signal Specification : SignalSpecification
  Signal Specification1 : SignalSpecification
  Signal Specification2 : SignalSpecification
  compute dependent gains : mach_lib/compute dependent gains
  params : Outport
  wires:
  Constant1/1 -> compute dependent gains/6
  Constant6/1 -> compute dependent gains/5
  Signal Specification2/1 -> compute dependent gains/4, Bus Creator/7  "kf"
  Bus Selector/2 -> Signal Specification1/1  "<MACH_pqr_Ki>"
  Bus Selector/1 -> Signal Specification/1  "<MACH_pqr_Kb>"
  gain_bus/1 -> Bus Selector/1
  compute dependent gains/4 -> Bus Creator/6  "x0"
  Bus Selector/3 -> compute dependent gains/3  "<MACH_pqr_Kaw>"
  compute dependent gains/2 -> Bus Creator/4  "ki_trim"
  compute dependent gains/1 -> Bus Creator/3  "kc"
  Bus Creator/1 -> params/1
  Signal Specification/1 -> Bus Creator/1, compute dependent gains/2  "kb"
  Signal Specification1/1 -> Bus Creator/2, compute dependent gains/1  "ki"
  compute dependent gains/3 -> Bus Creator/5  "kaw"
  Bus Selector/4 -> Signal Specification2/1  "<MACH_pqr_Kf>"

== system mach_lib/claw_main/input processing/set control parameters/set rate di params ==
  full_surf : Inport
  aero_env_est : Inport  Port=2
  Bus Creator1 : BusCreator  Inputs=7
  Bus Selector1 : BusSelector  OutputSignals=full_surf_ulim,full_surf_llim
  Bus Selector2 : BusSelector  OutputSignals=full_surf_urlim,full_surf_lrlim
  Bus Selector3 : BusSelector  OutputSignals=qbar
  Constant5 : Constant  Value=MACH.pqr_wght_cv
  Relay : Relay  OnSwitchValue=aero_surf_qbar_on  OffSwitchValue=aero_surf_qbar_off  OnOutputValue=0  OffOutputValue=1
  Selector{1..2,5..6} (4 alike) : Selector  Elements=MACH.pqr_u_idx  InputPortWidth=MACH.num_u
  fix aero surfs when low qbar : Subsystem
  limit schedule : model_lib/no limit schedule
  select u_pref : Subsystem
  rate_params : Outport
  wires:
  Relay/1 -> select u_pref/1(low_qbar), fix aero surfs when low qbar/3(low_qbar)
  Bus Selector3/1 -> Relay/1  "<qbar>"
  Constant5/1 -> Bus Creator1/7  "wght_cv"
  Bus Selector2/2 -> Selector2/1  "<full_surf_lrlim>"
  Bus Selector2/1 -> Selector1/1  "<full_surf_urlim>"
  limit schedule/2 -> fix aero surfs when low qbar/2(pqr_u_llim_in)
  limit schedule/1 -> fix aero surfs when low qbar/1(pqr_u_ulim_in)
  fix aero surfs when low qbar/2(pqr_u_llim) -> Bus Creator1/4  "u_llim"
  fix aero surfs when low qbar/1(pqr_u_ulim) -> Bus Creator1/3  "u_ulim"
  Selector2/1 -> Bus Creator1/2  "u_lrlim"
  Selector1/1 -> Bus Creator1/1  "u_urlim"
  aero_env_est/1 -> Bus Selector3/1, limit schedule/3, select u_pref/2(aero_env_est)
  Selector5/1 -> limit schedule/1
  Bus Selector1/2 -> Selector6/1  "<full_surf_llim>"
  Bus Selector1/1 -> Selector5/1  "<full_surf_ulim>"
  Selector6/1 -> limit schedule/2
  full_surf/1 -> select u_pref/3(full_surf), Bus Selector2/1, Bus Selector1/1
  Bus Creator1/1 -> rate_params/1
  select u_pref/1(u_pref) -> fix aero surfs when low qbar/4(pqr_u_pref), Bus Creator1/5  "u_pref"
  select u_pref/2(wght_u_pref) -> Bus Creator1/6  "wght_u_pref"

== system mach_lib/claw_main/input processing/set control parameters/set vel desdyn params ==
  gain_bus : Inport
  Bus Creator : BusCreator  Inputs=7
  Bus Selector : BusSelector  OutputSignals=MACH_vel_Kb,MACH_vel_Ki,MACH_vel_Kaw,MACH_vel_Kf
  Constant1 : Constant  Value=MACH_vel_cvdnom_IC
  Constant6 : Constant  Value=MACH_vel_IC
  Signal Specification : SignalSpecification
  Signal Specification1 : SignalSpecification
  Signal Specification2 : SignalSpecification
  compute dependent gains : mach_lib/compute dependent gains
  params : Outport
  wires:
  Constant1/1 -> compute dependent gains/6
  Constant6/1 -> compute dependent gains/5
  compute dependent gains/4 -> Bus Creator/6  "x0"
  Signal Specification2/1 -> Bus Creator/7  "kf"
  Signal Specification1/1 -> Bus Creator/2, compute dependent gains/1  "ki"
  Signal Specification/1 -> compute dependent gains/2, Bus Creator/1  "kb"
  gain_bus/1 -> Bus Selector/1
  Bus Selector/3 -> compute dependent gains/3  "<MACH_vel_Kaw>"
  compute dependent gains/2 -> Bus Creator/4  "ki_trim"
  compute dependent gains/1 -> Bus Creator/3  "kc"
  Bus Creator/1 -> params/1
  Bus Selector/1 -> Signal Specification/1  "<MACH_vel_Kb>"
  Bus Selector/2 -> Signal Specification1/1  "<MACH_vel_Ki>"
  compute dependent gains/3 -> Bus Creator/5  "kaw"
  Bus Selector/4 -> compute dependent gains/4, Signal Specification2/1  "<MACH_vel_Kf>"

== system mach_lib/claw_main/rate_loops/B matrix comp/cvd_def_nom ==
  x : Inport
  u : Inport  Port=2
  xdot : Inport  Port=3
  Selector : Selector  Elements=MACH.pqr_idx  InputPortWidth=MACH.num_x
  Terminator : Terminator
  Terminator1 : Terminator
  cvd : Outport
  wires:
  x/1 -> Terminator1/1
  u/1 -> Terminator/1
  Selector/1 -> cvd/1
  xdot/1 -> Selector/1

== system mach_lib/claw_main/rate_loops/B matrix comp/cvd_def_pert ==
  x : Inport
  u : Inport  Port=2
  xdot : Inport  Port=3
  Selector : Selector  Elements=MACH.pqr_idx  InputPortWidth=MACH.num_x
  Terminator : Terminator
  Terminator1 : Terminator
  cvd : Outport
  wires:
  x/1 -> Terminator1/1
  u/1 -> Terminator/1
  Selector/1 -> cvd/1
  xdot/1 -> Selector/1

== system mach_lib/claw_main/rate_loops/B matrix comp/pert insert ==
  X_nom : Inport
  U_nom : Inport  Port=2
  D_pert : Inport  Port=3
  Assignment : Assignment  Elements=MACH.pqr_u_idx  OutputInitialize=Initialize using input (U1)
  X_pert : Outport
  U_pert : Outport  Port=2
  wires:
  U_nom/1 -> Assignment/1
  X_nom/1 -> X_pert/1
  Assignment/1 -> U_pert/1
  D_pert/1 -> Assignment/2

== system mach_lib/claw_main/rate_loops/B matrix comp/pert_comp ==
  col : Inport
  d_nom : Inport  Port=2
  params : Inport  Port=3
  Bus Selector : BusSelector  OutputSignals=u_ulim,u_llim
  Constant2 : Constant  Value=diag(MACH.pqr_u_pert)
  pick +/- pert : mach_lib/pick +//- pert  num_u=MACH.pqr_num_u
  d_pert : Outport
  d_div : Outport  Port=2
  wires:
  Bus Selector/2 -> pick +/- pert/4  "<u_llim>"
  params/1 -> Bus Selector/1
  Bus Selector/1 -> pick +/- pert/3  "<u_ulim>"
  d_nom/1 -> pick +/- pert/2
  col/1 -> pick +/- pert/1
  pick +/- pert/2 -> d_div/1  "scalar pert value"
  pick +/- pert/1 -> d_pert/1
  Constant2/1 -> pick +/- pert/5

== system mach_lib/claw_main/rate_loops/allocation/RCS allocation ==
  Bmat : Inport
  rcs_cmd_old : Inport  Port=2
  cvd_des : Inport  Port=3
  params : Inport  Port=4
  Bus Selector : BusSelector  OutputSignals=wght_cv,u_ulim,u_llim
  Constant : Constant  Value=[1 1 1]
  Constant1 : Constant  Value=MACH.pqr_rcs_use
  Constant2 : Constant  Value=rcs_cvddes_thresh
  Embedded MATLAB Function : Stateflow chart
  Sum5 : Sum  Inputs=+-|  SaturateOnIntegerOverflow=on  InputSameDT=on
  Terminator{,1..3} (4 alike) : Terminator
  rcs_cmd : Outport
  cvd_extra : Outport  Port=2
  wires:
  Constant/1 -> Embedded MATLAB Function/2(wght_cv)
  Bus Selector/1 -> Terminator1/1  "<wght_cv>"
  Constant1/1 -> Embedded MATLAB Function/7(rcs_use_in)
  Bus Selector/2 -> Embedded MATLAB Function/3(ulim)  "<u_ulim>"
  Bus Selector/3 -> Embedded MATLAB Function/4(llim)  "<u_llim>"
  Constant2/1 -> Embedded MATLAB Function/6(err_thresh)
  rcs_cmd_old/1 -> Terminator/1
  Embedded MATLAB Function/4(cvd_actual) -> Sum5/1
  Embedded MATLAB Function/2(minerr) -> Terminator2/1
  Embedded MATLAB Function/1(rcs_cmd) -> rcs_cmd/1
  Bmat/1 -> Embedded MATLAB Function/1(Bmat)
  Sum5/1 -> cvd_extra/1
  cvd_des/1 -> Embedded MATLAB Function/5(cvd_des), Sum5/2
  params/1 -> Bus Selector/1
  Embedded MATLAB Function/3(scale) -> Terminator3/1

== system mach_lib/claw_main/rate_loops/allocation/config_di ==
  cvd_nom : Inport
  Bmat : Inport  Port=2
  d_old : Inport  Port=3
  d_nom : Inport  Port=4
  cvd_des : Inport  Port=5
  params : Inport  Port=6
  di_smn : mach_lib/di_smn
  d_cmd : Outport
  cvd_extra : Outport  Port=2
  lambda : Outport  Port=3
  solve_dat : Outport  Port=4
  wires:
  di_smn/4 -> solve_dat/1
  di_smn/3 -> lambda/1
  di_smn/2 -> cvd_extra/1
  di_smn/1 -> d_cmd/1
  params/1 -> di_smn/6
  cvd_des/1 -> di_smn/5
  d_nom/1 -> di_smn/4
  d_old/1 -> di_smn/3
  Bmat/1 -> di_smn/2
  cvd_nom/1 -> di_smn/1

== system mach_lib/claw_main/rate_loops/allocation/param select rcs ==
  params_all : Inport
  Bus Creator1 : BusCreator  Inputs=7
  Bus Selector : BusSelector  OutputSignals=u_ulim,u_llim,u_urlim,u_lrlim,u_pref,wght_u_pref,wght_cv
  Selector{,1..5} (6 alike) : Selector  Elements=idx  InputPortWidth=MACH.pqr_num_u
  params : Outport
  wires:
  Bus Selector/7 -> Bus Creator1/7  "<wght_cv>"
  Selector5/1 -> Bus Creator1/6  "wght_u_pref"
  Selector4/1 -> Bus Creator1/5  "u_pref"
  Selector1/1 -> Bus Creator1/2  "u_llim"
  Selector/1 -> Bus Creator1/1  "u_ulim"
  Selector2/1 -> Bus Creator1/3  "u_urlim"
  Selector3/1 -> Bus Creator1/4  "u_lrlim"
  params_all/1 -> Bus Selector/1
  Bus Selector/1 -> Selector/1  "<u_ulim>"
  Bus Selector/2 -> Selector1/1  "<u_llim>"
  Bus Selector/3 -> Selector2/1  "<u_urlim>"
  Bus Selector/4 -> Selector3/1  "<u_lrlim>"
  Bus Selector/5 -> Selector4/1  "<u_pref>"
  Bus Selector/6 -> Selector5/1  "<wght_u_pref>"
  Bus Creator1/1 -> params/1

== system mach_lib/claw_main/rate_loops/allocation/param select smn ==
  params_all : Inport
  Bus Creator1 : BusCreator  Inputs=7
  Bus Selector : BusSelector  OutputSignals=u_ulim,u_llim,u_urlim,u_lrlim,u_pref,wght_u_pref,wght_cv
  Selector{,1..5} (6 alike) : Selector  Elements=idx  InputPortWidth=MACH.pqr_num_u
  params : Outport
  wires:
  Bus Creator1/1 -> params/1
  Bus Selector/6 -> Selector5/1  "<wght_u_pref>"
  Bus Selector/5 -> Selector4/1  "<u_pref>"
  Bus Selector/4 -> Selector3/1  "<u_lrlim>"
  Bus Selector/3 -> Selector2/1  "<u_urlim>"
  Bus Selector/2 -> Selector1/1  "<u_llim>"
  Bus Selector/1 -> Selector/1  "<u_ulim>"
  params_all/1 -> Bus Selector/1
  Selector3/1 -> Bus Creator1/4  "u_lrlim"
  Selector2/1 -> Bus Creator1/3  "u_urlim"
  Selector/1 -> Bus Creator1/1  "u_ulim"
  Selector1/1 -> Bus Creator1/2  "u_llim"
  Selector4/1 -> Bus Creator1/5  "u_pref"
  Selector5/1 -> Bus Creator1/6  "wght_u_pref"
  Bus Selector/7 -> Bus Creator1/7  "<wght_cv>"

== system mach_lib/claw_main/rate_loops/select rate cmd/get direct cmd ==
  signal_bus : Inport
  Bus Selector1 : BusSelector  OutputSignals=cmd_bus.autopilot_cmd,mode_sw.full_surf_cmd_sw,full_surf.full_surf_cmd
  Demux2 : Demux  Outputs=[ 3 1 ]
  Gain1 : Gain  Gain=MACH.throt_mixer
  Multiport Switch2 : MultiPortSwitch  Inputs=2  zeroidx=on
  Mux2 : Mux  Inputs=2
  throttle : Selector  Elements=MACH.throttle_idx  InputPortWidth=MACH.num_u
  direct_cmd : Outport
  wires:
  Multiport Switch2/1 -> Mux2/2
  throttle/1 -> Multiport Switch2/3
  Bus Selector1/3 -> throttle/1  "<full_surf_cmd>"
  Gain1/1 -> Multiport Switch2/2
  Bus Selector1/2 -> Multiport Switch2/1  "<full_surf_cmd_sw>"
  Bus Selector1/1 -> Demux2/1  "<autopilot_cmd>"
  signal_bus/1 -> Bus Selector1/1
  Mux2/1 -> direct_cmd/1
  Demux2/2 -> Gain1/1
  Demux2/1 -> Mux2/1

== system mach_lib/claw_main/state est/process sensors/compute dc_fltpath ==
  NEh_dot_fltpath : Inport
  Gain : Gain  Gain=repmat([1 1 -1],3,1)
  Gain1 : Gain  Gain=[1 1 -1]
  Reshape : simulink/Math Operations/Reshape  OutputDimensionality=Customize  OutputDimensions=[3 3]
  Terminator : Terminator
  vec2dc : utility_lib/vec2dc
  dc_fltpath : Outport
  wires:
  NEh_dot_fltpath/1 -> Gain1/1
  Gain/1 -> dc_fltpath/1
  vec2dc/2 -> Terminator/1
  Gain1/1 -> vec2dc/1
  Reshape/1 -> Gain/1
  vec2dc/1 -> Reshape/1

== system mach_lib/claw_main/state est/process sensors/navigation complementary filter ==
  NEh nav : Inport
  NEh dot : Inport  Port=2
  Gain1 : Gain  Gain=MACH.K_velpos  SaturateOnIntegerOverflow=on
  Sum1 : Sum  Inputs=|+-  SaturateOnIntegerOverflow=on
  Sum2 : Sum  Inputs=++|  SaturateOnIntegerOverflow=on  InputSameDT=on
  integration1 : DiscreteIntegrator  SampleTime=-1  ICPrevOutput=DiscIntNeverNeededParam  ICPrevScaledInput=DiscIntNeverNeededParam
  NEh_fil : Outport
  wires:
  Sum1/1 -> Gain1/1
  integration1/1 -> Sum1/2, NEh_fil/1
  Sum2/1 -> integration1/1
  Gain1/1 -> Sum2/2
  NEh nav/1 -> Sum1/1
  NEh dot/1 -> Sum2/1

== system mach_lib/claw_main/state est/process sensors/select e sign ==
  e in : Inport
  e_past : Inport  Port=2
  Dot Product : simulink/Math Operations/Dot Product  InputSameDT=on  OutDataType=sfix(16)  OutScaling=2^-10  DoSatur=off
  Gain : Gain  Gain=-1  SaturateOnIntegerOverflow=on
  Switch : Switch  SaturateOnIntegerOverflow=on
  e out : Outport
  wires:
  e in/1 -> Dot Product/1, Switch/1, Gain/1
  Dot Product/1 -> Switch/2
  Gain/1 -> Switch/3
  Switch/1 -> e out/1
  e_past/1 -> Dot Product/2

== system mach_lib/claw_main/state est/process sensors/wait for valid nav ==
  latlonh : Inport
  nav_ok : Inport  Port=2
  Switch3 : Switch  Threshold=0.5  SaturateOnIntegerOverflow=on
  Unit Delay1 : UnitDelay  Orientation=left  SampleTime=-1
  LLh_0 : Outport
  nav_valid : Outport  Port=2
  wires:
  Unit Delay1/1 -> Switch3/1
  Switch3/1 -> LLh_0/1, Unit Delay1/1
  latlonh/1 -> Switch3/3
  nav_ok/1 -> Switch3/2, nav_valid/1
